simulink model "all1"  (R2016b)
settings: Solver=VariableStepAuto  StartTime=0.0  StopTime=20  RelTol=1e-3
libraries: simulink x1
settings Model: Creator=lenovo  LastModifiedBy=lenovo

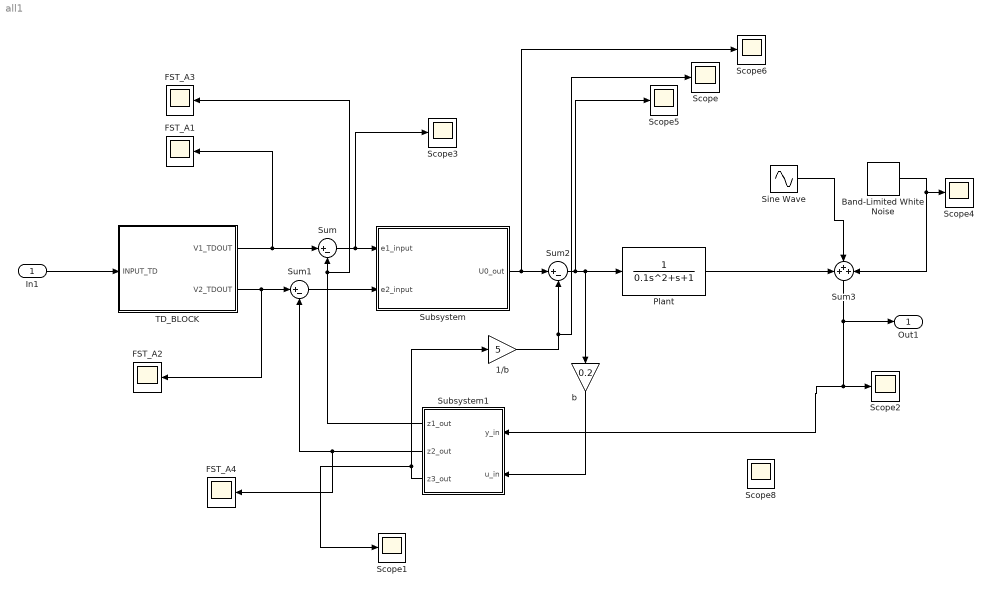
== system all1 ==
  In1 : Inport
  1/b : Gain  Gain=5
  Band-Limited White Noise : simulink/Sources/Band-Limited White Noise  Cov=[0.0]  Ts=0.1  seed=[23341]
  FST_A{1..4} (4 alike) : Scope
  Plant : TransferFcn  Denominator=[0.1 1 1]
  Scope{,1..6,8} (8 alike) : Scope
  Sine Wave : Sin  Frequency=2  SampleTime=0
  Subsystem : Subsystem
  Subsystem1 : Subsystem
  Sum : Sum  Inputs=|+-
  Sum1 : Sum  Inputs=|+-
  Sum2 : Sum  Inputs=|+-
  Sum3 : Sum  Inputs=+++
  TD_BLOCK : Subsystem
  b : Gain  Gain=0.2
  Out1 : Outport
  wires:
  In1/1 -> TD_BLOCK/1(INPUT_TD)
  TD_BLOCK/1(V1_TDOUT) -> Sum/1, FST_A1/1
  TD_BLOCK/2(V2_TDOUT) -> Sum1/1, FST_A2/1
  Subsystem/1(U0_out) -> Scope6/1, Sum2/1
  Sum/1 -> Subsystem/1(e1_input), Scope3/1
  Sum1/1 -> Subsystem/2(e2_input)
  Subsystem1/1(z1_out) -> FST_A3/1, Sum/2
  Subsystem1/3(z3_out) -> Scope1/1, 1/b/1
  1/b/1 -> Scope/1, Sum2/2
  Sum2/1 -> Scope5/1, b/1, Plant/1
  b/1 -> Subsystem1/2(u_in)
  Subsystem1/2(z2_out) -> FST_A4/1, Sum1/2
  Sum3/1 -> Out1/1, Subsystem1/1("y_in "), Scope2/1
  Sine Wave/1 -> Sum3/2
  Band-Limited White Noise/1 -> Sum3/3, Scope4/1
  Plant/1 -> Sum3/1

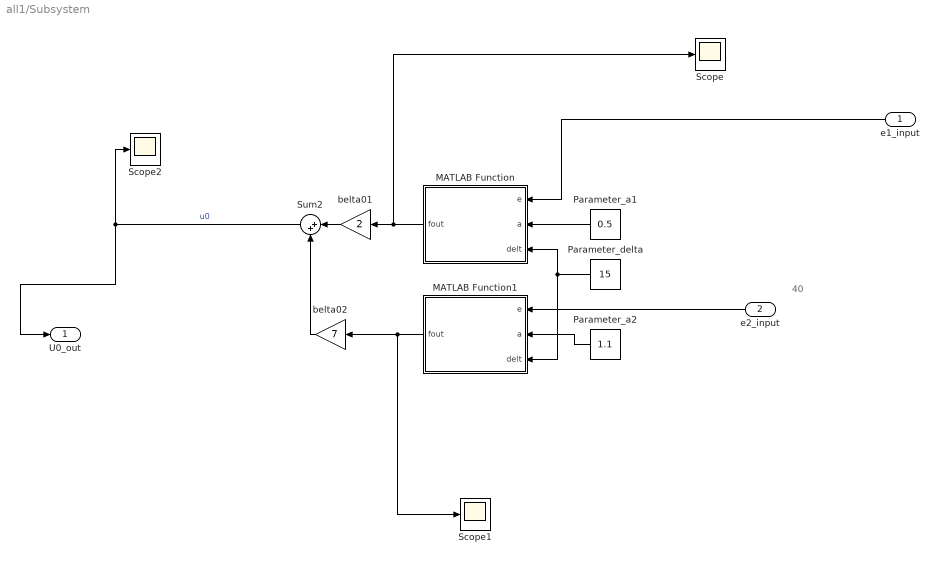
== system all1/Subsystem ==
  note: 40
  e1_input : Inport
  e2_input : Inport  Port=2
  MATLAB Function : MATLAB Function  TreatAsAtomicUnit=on
  MATLAB Function1 : MATLAB Function  TreatAsAtomicUnit=on
  Parameter_a1 : Constant  Value=0.5
  Parameter_a2 : Constant  Value=1.1
  Parameter_delta : Constant  Value=15
  Scope : Scope
  Scope1 : Scope
  Scope2 : Scope
  Sum2 : Sum  Inputs=|++
  belta01 : Gain  Gain=2
  belta02 : Gain  Gain=7
  U0_out : Outport
  wires:
  MATLAB Function/1(fout) -> Scope/1, belta01/1
  MATLAB Function1/1(fout) -> Scope1/1, belta02/1
  belta01/1 -> Sum2/1
  Parameter_a2/1 -> MATLAB Function1/2(a)
  belta02/1 -> Sum2/2
  Sum2/1 -> U0_out/1, Scope2/1  "u0"
  Parameter_a1/1 -> MATLAB Function/2(a)
  Parameter_delta/1 -> MATLAB Function/3(delt), MATLAB Function1/3(delt)
  e1_input/1 -> MATLAB Function/1(e)
  e2_input/1 -> MATLAB Function1/1(e)

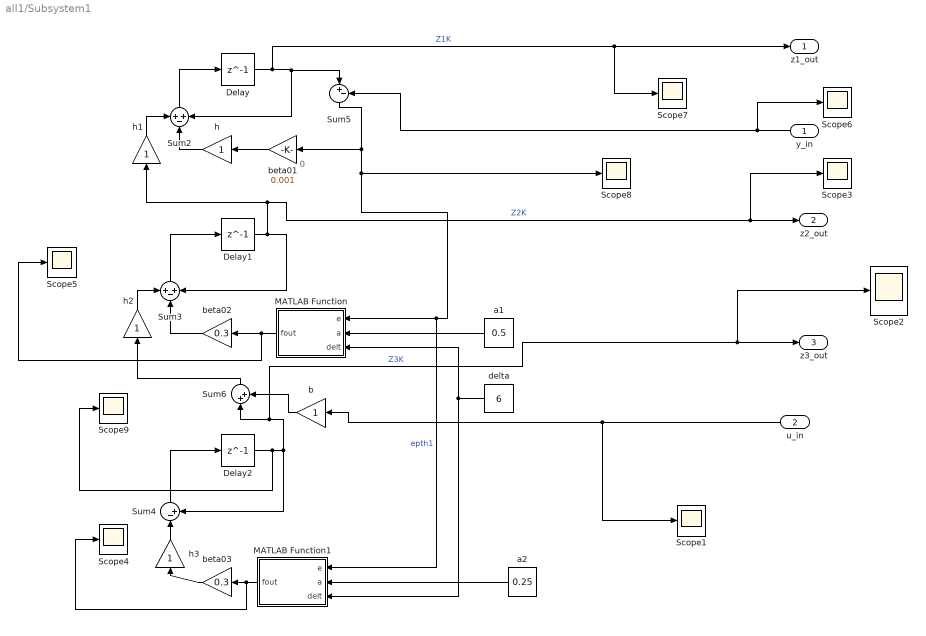
== system all1/Subsystem1 ==
  note: 0
  "y_in " : Inport
  u_in : Inport  Port=2
  Delay : Delay  DelayLength=1
  Delay1 : Delay  DelayLength=1
  Delay2 : Delay  DelayLength=1
  MATLAB Function : MATLAB Function  TreatAsAtomicUnit=on
  MATLAB Function1 : MATLAB Function  TreatAsAtomicUnit=on
  Scope{1..9} (9 alike) : Scope
  Sum2 : Sum  Inputs=+-+
  Sum3 : Sum  Inputs=+-+
  Sum4 : Sum  Inputs=|-+
  Sum5 : Sum  Inputs=|+-
  Sum6 : Sum  Inputs=|++
  a1 : Constant  Value=0.5
  a2 : Constant  Value=0.25
  b : Gain
  beta01 : Gain  Gain=0.001
  beta02 : Gain  Gain=0.3
  beta03 : Gain  Gain=0.3
  delta : Constant  Value=6
  h{,1..3} (4 alike) : Gain
  z1_out : Outport
  z2_out : Outport  Port=2
  z3_out : Outport  Port=3
  wires:
  h3/1 -> Sum4/1
  Delay2/1 -> Scope9/1, Sum4/2, Scope2/1, z3_out/1, Sum6/1  "Z3K"
  "y_in "/1 -> Scope6/1, Sum5/2
  beta01/1 -> h/1
  b/1 -> Sum6/2
  delta/1 -> MATLAB Function/3(delt), MATLAB Function1/3(delt)
  h/1 -> Sum2/2
  Delay1/1 -> Scope3/1, z2_out/1, h1/1, Sum3/3  "Z2K"
  Sum4/1 -> Delay2/1
  h1/1 -> Sum2/1
  beta03/1 -> h3/1
  h2/1 -> Sum3/1
  a1/1 -> MATLAB Function/2(a)
  a2/1 -> MATLAB Function1/2(a)
  Delay/1 -> Scope7/1, z1_out/1, Sum5/1, Sum2/3  "Z1K"
  Sum2/1 -> Delay/1
  MATLAB Function/1(fout) -> Scope5/1, beta02/1
  u_in/1 -> Scope1/1, b/1
  Sum6/1 -> h2/1
  Sum5/1 -> Scope8/1, MATLAB Function1/1(e), MATLAB Function/1(e), beta01/1  "epth1"
  beta02/1 -> Sum3/2
  MATLAB Function1/1(fout) -> Scope4/1, beta03/1
  Sum3/1 -> Delay1/1

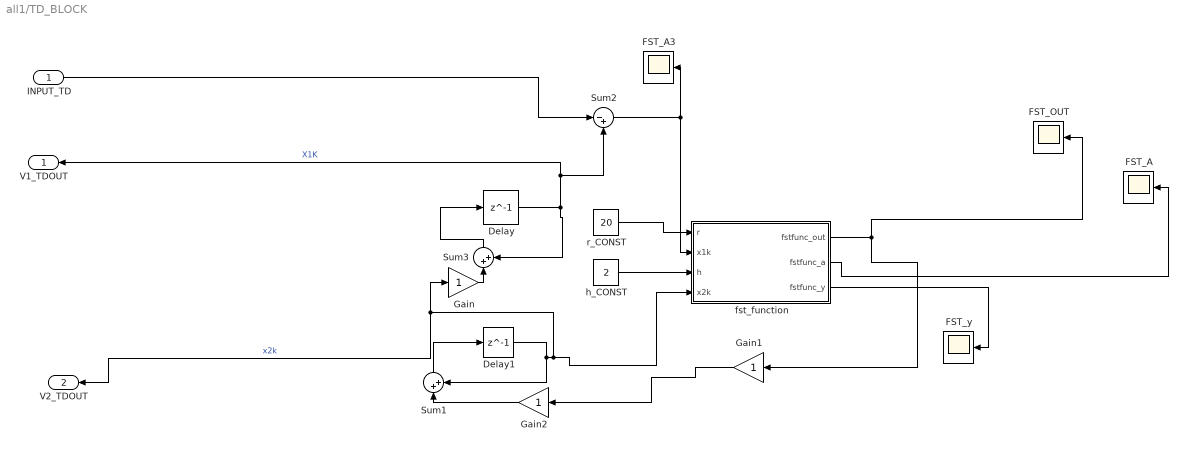
== system all1/TD_BLOCK ==
  INPUT_TD : Inport
  Delay : Delay  DelayLength=1  InitialCondition=0
  Delay1 : Delay  DelayLength=1
  FST_A : Scope
  FST_A3 : Scope
  FST_OUT : Scope
  FST_y : Scope
  Gain : Gain
  Gain1 : Gain
  Gain2 : Gain
  Sum1 : Sum  Inputs=|++
  Sum2 : Sum  Inputs=|-+
  Sum3 : Sum  Inputs=|++
  fst_function : Subsystem
  h_CONST : Constant  Value=2
  r_CONST : Constant  Value=20
  V1_TDOUT : Outport
  V2_TDOUT : Outport  Port=2
  wires:
  Sum1/1 -> Delay1/1
  INPUT_TD/1 -> Sum2/1
  Sum2/1 -> FST_A3/1, fst_function/2(x1k)
  r_CONST/1 -> fst_function/1(r)
  h_CONST/1 -> fst_function/3(h)
  Delay1/1 -> Sum1/2, V2_TDOUT/1, Gain/1, fst_function/4(x2k)  "x2k"
  Delay/1 -> Sum3/2, V1_TDOUT/1, Sum2/2  "X1K"
  fst_function/1(fstfunc_out) -> Gain1/1, FST_OUT/1
  Gain1/1 -> Gain2/1
  Gain2/1 -> Sum1/1
  fst_function/3(fstfunc_y) -> FST_y/1
  Gain/1 -> Sum3/1
  Sum3/1 -> Delay/1
  fst_function/2(fstfunc_a) -> FST_A/1

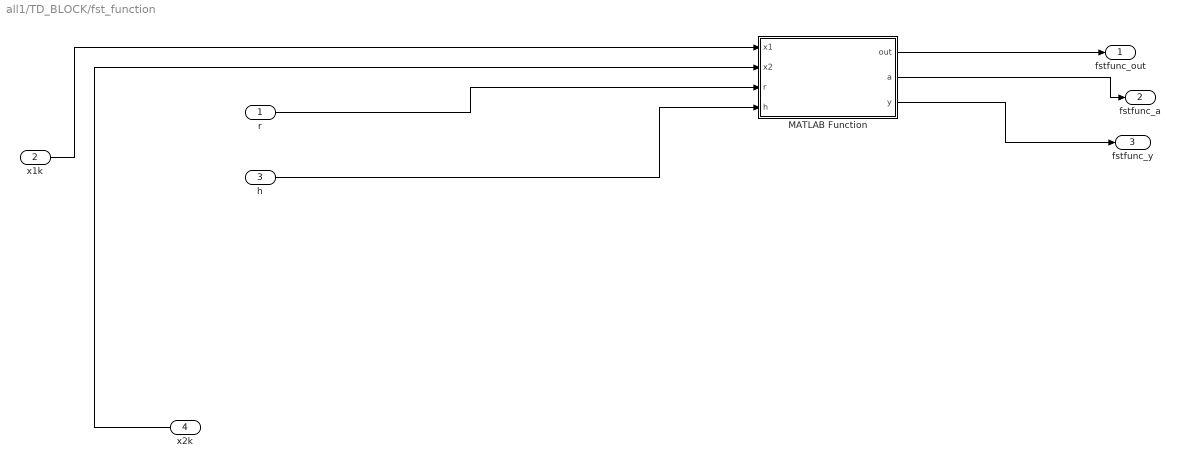
== system all1/TD_BLOCK/fst_function ==
  r : Inport
  x1k : Inport  Port=2
  h : Inport  Port=3
  x2k : Inport  Port=4
  MATLAB Function : MATLAB Function  TreatAsAtomicUnit=on
  fstfunc_out : Outport
  fstfunc_a : Outport  Port=2
  fstfunc_y : Outport  Port=3
  wires:
  x2k/1 -> MATLAB Function/2(x2)
  r/1 -> MATLAB Function/3(r)
  h/1 -> MATLAB Function/4(h)
  MATLAB Function/1(out) -> fstfunc_out/1
  x1k/1 -> MATLAB Function/1(x1)
  MATLAB Function/2(a) -> fstfunc_a/1
  MATLAB Function/3(y) -> fstfunc_y/1

== matlab function all1/Subsystem/MATLAB Function ==
  data: e input; fout output; a input; delt input
function fout= falfcn(e,a,delt)
if abs(e)>delt
    fal=(abs(e))^a*sign(e);
else
    fal=delt^(1-a);
    fal=e/fal;
end
fout=fal;

end

== matlab function all1/TD_BLOCK/fst_function/MATLAB Function ==
  data: x1 input; out output; x2 input; r input; h input; a output; y output
function [out,a,y] = fst_test(x1,x2,r,h)
d=r*h;
d0=d*h;
y=x1+h*x2;
a0=sqrt(d*d+8*r*abs(y));
absy=abs(y);
if absy>d0
    a=x2+0.5*a0-0.5*d;
else
    a=x2+y/h;
end
absa=abs(a);
if absa<=d0
    out=-r*a/d;
else
    out=-r*sign(a);
end

end

== matlab function all1/Subsystem/MATLAB Function1 ==
  data: e input; fout output; a input; delt input
function fout= falfcn(e,a,delt)
if abs(e)>delt
    fal=(abs(e))^a*sign(e);
else
    fal=delt^(1-a);
    fal=e/fal;
end
fout=fal;

end

== matlab function all1/Subsystem1/MATLAB Function ==
  data: e input; fout output; a input; delt input
function fout= falfcn(e,a,delt)
if abs(e)>delt
    fal=(abs(e))^a*sign(e);
else
    fal=delt^(1-a);
    fal=e/fal;
end
fout=fal;

end

== matlab function all1/Subsystem1/MATLAB Function1 ==
  data: e input; fout output; a input; delt input
function fout= falfcn(e,a,delt)
if abs(e)>delt
    fal=(abs(e))^a*sign(e);
else
    fal=delt^(1-a);
    fal=e/fal;
end
fout=fal;

end
